simulink model "observer_with_state_feedback_integrator"  (R2020b)
settings: Solver=VariableStepAuto  StartTime=0.0  StopTime=25  RelTol=1e-3
values from neighbouring files (symbols this model uses):
  A = [0 1 0 0 ... (first row only)    [eight_state_feedback.m]    (also in eleven_full_order_observer.m; observerfornonlinearsystem.m; seven_controllability_and_observebility.m; state_feedback_integrator.m)
  B = [0; 0; 0; 1]    [eight_state_feedback.m]    (also in eleven_full_order_observer.m; observerfornonlinearsystem.m; seven_controllability_and_observebility.m; state_feedback_integrator.m)
  C = [1 0 0 0]    [eight_state_feedback.m]    (also in eleven_full_order_observer.m; observerfornonlinearsystem.m; seven_controllability_and_observebility.m; state_feedback_integrator.m)
  K1 = K ( 1 : rA )    [state_feedback_integrator.m]
  K2 = K ( rA + 1 : rA + rC )    [state_feedback_integrator.m]
  L = L_transpose'    [eleven_full_order_observer.m]    (also in observerfornonlinearsystem.m; state_feedback_with_observer_for_nonlinear_system.m)
settings Model: Creator=Alireza  LastModifiedBy=Alireza

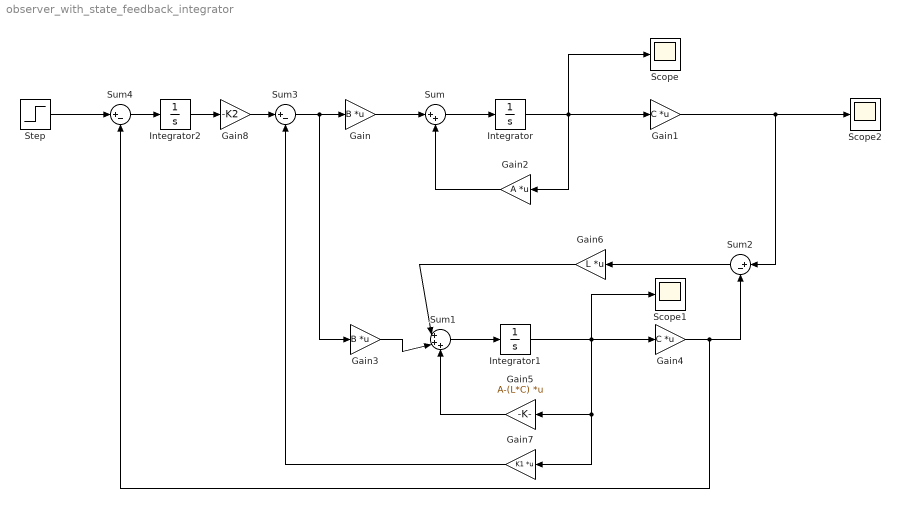
== system observer_with_state_feedback_integrator ==
  Gain : Gain  Gain=B  Multiplication=Matrix(K*u)
  Gain1 : Gain  Gain=C  Multiplication=Matrix(K*u)
  Gain2 : Gain  Gain=A  Multiplication=Matrix(K*u)
  Gain3 : Gain  Gain=B  Multiplication=Matrix(K*u)
  Gain4 : Gain  Gain=C  Multiplication=Matrix(K*u)
  Gain5 : Gain  Gain=A-(L*C)  Multiplication=Matrix(K*u)
  Gain6 : Gain  Gain=L  Multiplication=Matrix(K*u)
  Gain7 : Gain  Gain=K1  Multiplication=Matrix(K*u)
  Gain8 : Gain  Gain=-K2
  Integrator : Integrator  InitialCondition=1
  Integrator1 : Integrator  InitialCondition=-2
  Integrator2 : Integrator
  Scope : Scope
  Scope1 : Scope
  Scope2 : Scope
  Step : Step  SampleTime=0
  Sum : Sum  Inputs=|++
  Sum1 : Sum  Inputs=|+++
  Sum2 : Sum  Inputs=|+-
  Sum3 : Sum  Inputs=|+-
  Sum4 : Sum  Inputs=|+-
  wires:
  Gain/1 -> Sum/1
  Gain3/1 -> Sum1/2
  Gain6/1 -> Sum1/1
  Gain5/1 -> Sum1/3
  Sum1/1 -> Integrator1/1
  Integrator1/1 -> Scope1/1, Gain4/1, Gain7/1, Gain5/1
  Sum2/1 -> Gain6/1
  Integrator/1 -> Scope/1, Gain1/1, Gain2/1
  Sum/1 -> Integrator/1
  Gain2/1 -> Sum/2
  Sum3/1 -> Gain3/1, Gain/1
  Step/1 -> Sum4/1
  Gain1/1 -> Sum2/1, Scope2/1
  Gain8/1 -> Sum3/1
  Integrator2/1 -> Gain8/1
  Sum4/1 -> Integrator2/1
  Gain4/1 -> Sum2/2, Sum4/2
  Gain7/1 -> Sum3/2
